simulink model "wlan_phy_tx_pmd"  (Simulink 7.8)
settings: Solver=ode45  StartTime=0.0  StopTime=17e3  RelTol=1e-3
PostLoadFcn:
  | wlan_phy_tx_init
InitFcn:
  | wlan_phy_tx_init
StartFcn:
  | wlan_phy_tx_init
values from neighbouring files (symbols this model uses):
  interleave_64QAM_addr = interleave_64QAM + 2*floor(interleave_64QAM/6)    [wlan_phy_tx_init.m]
  MAX_NUM_BYTES = 4096    [wlan_phy_tx_init.m]
  MAX_NUM_SC = 64    [wlan_phy_tx_init.m]
  Preamble_IQ = PLCP_Preamble.Preamble_t    [wlan_phy_tx_init.m]
undefined symbols (not defined in the file or in its folder): gcbh, interleave_16QAM, interleave_bpsk, interleave_QPSK, Mod_Constellation_16QAM, Mod_Constellation_64QAM, Mod_Constellation_BPSK, Mod_Constellation_QPSK, xlBlockLoadCallback, xlGetNormalizedPeriod
libraries: xbsIndex_r4 x1023, xbsEDKLib_r4 x1
(part 1 of 8)
settings Model: Creator=murphpo  LastModifiedBy=murphpo
settings DebuggingCC: SolverPrmCheckMsg=none  InheritedTsInSrcMsg=none  UnconnectedInputMsg=none  UnconnectedOutputMsg=none  UnconnectedLineMsg=none

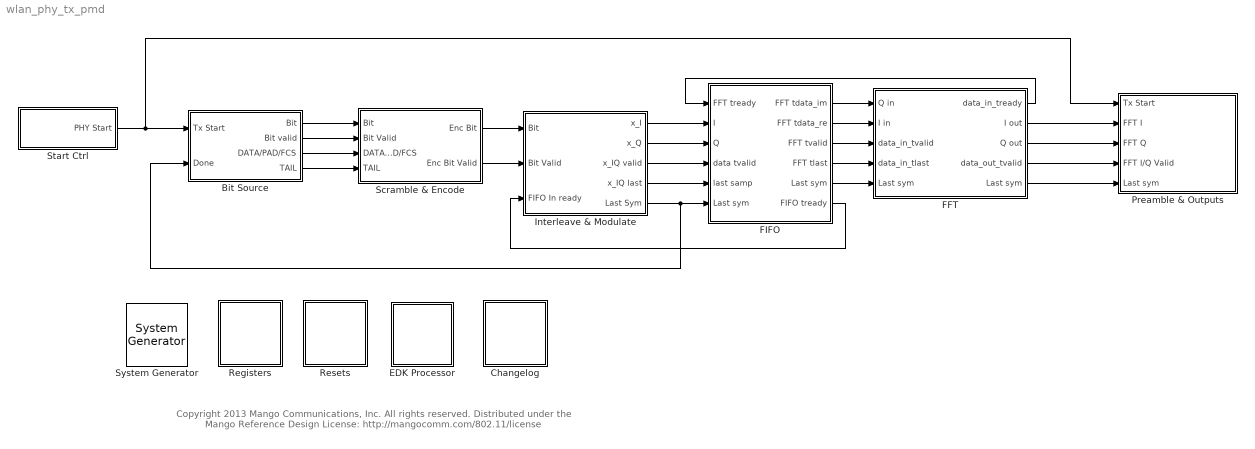
== system wlan_phy_tx_pmd ==
  note: Copyright 2013 Mango Communications, Inc. All rights reserved.
      |
      | Distributed under the Mango Reference Design License:
      | http://mangocomm.com/802.11/license
  " System Generator" : xbsIndex_r4/ System Generator  Tag=genX  xilinxfamily=virtex6  part=xc6vlx240t  speed=-2  package=ff1156  synthesis_tool=XST  clock_wrapper=Clock Enables  directory=./pcore_tx_v214  proj_type=Project Navigator  Synth_file=XST Defaults  Impl_file=ISE Defaults  testbench=off  simulink_period=1  sysclk_period=6.25  dcm_input_clock_period=10  incr_netlist=off  trim_vbits=Everywhere in SubSystem  dbl_ovrd=According to Block Masks  core_generation=According to Block Masks  run_coregen=off  deprecated_control=off  eval_field=0  block_type=sysgen
  Bit Source : Subsystem
  Changelog : Subsystem
  EDK Processor : Subsystem  LoadFcn=xlBlockLoadCallback(gcbh);  mask(Xilinx EDK Processor Block){mode=EDK pcore generation, xmp=, MemVisToProc=<qt bgcolor="#FFFFFF"><div><img src="S:/Xilinx/14.4/ISE_DS/ISE/sysgen/data/images/registerplus.gif"> &lt;&lt;Timing&gt;&gt;<br></div><div><img src="S:/Xilinx/14.4/ISE_DS/ISE/sysgen/data/images/registerplus.gif"> &lt;&lt;Config&gt;&gt;<br></div><div><img src="S:/Xilinx/14.4/ISE_DS/ISE/sysgen/data/images/registerplus.gif"> &lt;&lt;PKT_BUF_SEL&gt;&gt;<br></div><div><img src="S:/Xilinx/14.4/ISE_DS/ISE/sysgen/data/images/registerplus.gif"> &lt;&lt;Output_Scaling&gt;&gt;<br></div><div><img src="S:/Xilinx/14.4/ISE_DS/ISE/sysgen/data/images/registerplus.gif"> &lt;&lt;TX_START&gt;&gt;<br></div><div><img src="S:/Xilinx/14.4/ISE_DS/ISE/sysgen/data/images/registerplus.gif"> &lt;&lt;FFT_Config&gt;&gt;<br></div><div><img src="S:/Xilinx/14.4/ISE_DS/ISE/sysgen/data/images/registerplus.gif"> &lt;&lt;STATUS&gt;&gt;<br></div></qt>, AvailableMemories=<empty>, portInterfaceTable={'exposed'=>[],'portdir'=>[],'portname'=>[],'shortname'=>[]}, bus_type_sgadvanced=, bus_type=AXI, baseaddr=0x80000000, baseaddr_lock_sgadvanced=, baseaddr_lock=off, dual_clock_sgadvanced=, dual_clock=on, reg_readback_sgadvanced=, reg_readback=on, ucf_file=, inheritDeviceType_sgadvanced=, inheritDeviceType=off, elf_file=, codebug_sgadvanced=, codebug=on, clock_name=plb, internalPortList={}, resetPolarity=0, memxtable={'mladdr'=>[0.00000000000000000,1.00000000000000000,2.00000000000000000,3.00000000000000000,4.00000000000000000,5.00000000000000000,0.00000000000000000],'mlist'=>['wlan_phy_tx_pmd/Registers/From Register6','wlan_phy_tx_pmd/Registers/From Register5','wlan_phy_tx_pmd/Registers/From Register4','wlan_phy_tx_pmd/Registers/From Register3','wlan_phy_tx_pmd/Registers/From Register2','wlan_phy_tx_pmd/Registers/From Register1','wlan_phy_tx_pmd/Registers/To Register'],'mlname'=>['\\'Timing\\'','\\'Config\\'','\\'PKT_BUF_SEL\\'','\\'Output_Scaling\\'','\\'TX_START\\'','\\'FFT_Config\\'','\\'STATUS\\''],'mlstate'=>[0.00000000000000000,0.00000000000000000,0.00000000000000000,0.00000000000000000,0.00000000000000000,0.00000000000000000,0.00000000000000000]}, procinfo={}, memmapdirty=off, blockname=, xpsintstyle=default, has_advanced_control=0, sggui_pos=-1,-1,-1,-1, block_type=edkprocessor, block_version=2.7, sg_icon_stat=58,60,-1,-1,white,blue,0,07734,right,,[ ],[ ], sg_mask_display=|, sg_list_contents={'table'=>{'AvailableMemories'=>'popup(<empty>)'}}, sg_blockgui_xml=}
      mask sg_mask_display=|
      | fprintf('','COMMENT: begin icon graphics');
      | patch([0 58 58 0 0 ],[0 0 60 60 0 ],[0.77 0.82 0.91 ]);
      | plot([0 58 58 0 0 ],[0 0 60 60 0 ]);
      | patch([11.2 22.76 30.76 38.76 46.76 30.76 19.2 11.2 ],[38.88 38.88 46.88 38.88 46.88 46.88 46.88 38.88 ],[1 1 1 ]);
      | patch([19.2 30.76 22.76 11.2 19.2 ],[30.88 30.88 38.88 38.88 30.88 ],[0.931 0.946 0.973 ]);
      | patch([11.2 22.76 30.76 19.2 11.2 ],[22.88 22.88 30.88 30.88 22.88 ],[1 1 1 ]);
      | patch([19.2 46.76 38.76 30.76 22.76 11.2 19.2 ],[14.88 14.88 22.88 14.88 22.88 22.88 14.88 ],[0.931 0.946 0.973 ]);
      | fprintf('','COMMENT: end icon graphics');
      | fprintf('','COMMENT: begin icon text');
      | fprintf('','COMMENT: end icon text');
      mask prompts: mode "Configure Processor for"; xmp "XPS Project"; MemVisToProc ""; AvailableMemories "Available Memories"; portInterfaceTable ""; bus_type_sgadvanced ""; bus_type "Bus Type"; baseaddr "Base Address"; baseaddr_lock_sgadvanced ""; baseaddr_lock "Lock"; dual_clock_sgadvanced ""; dual_clock "Dual Clocks"; reg_readback_sgadvanced ""; reg_readback "Register Read-Back"; ucf_file "Constraint File"; inheritDeviceType_sgadvanced ""; inheritDeviceType "Inherit Device Type"; elf_file "Initial Program"; codebug_sgadvanced ""; codebug "Enable Co-Debug with Xilinx SDK (Beta)"; clock_name ""; internalPortList ""; resetPolarity ""; memxtable ""; procinfo ""; memmapdirty ""; blockname ""; xpsintstyle ""; has_advanced_control ""; sggui_pos ""; block_type ""; block_version ""; sg_icon_stat ""; sg_mask_display ""; sg_list_contents ""; sg_blockgui_xml ""
      mask help: Xilinx EDK Processor
      mask init:
      | try
      |   tmp_gcb = gcb;
      |   tmp_gcbh = gcbh;
      |   if (strcmp('SysGenIndex',get_param(bdroot(tmp_gcbh),'tag')) && ~isempty(regexp(bdroot(tmp_gcb), '^xbs', 'once')))
      |     return;
      |   end;
      |   xlMungeMaskParams;
      | 
      |   block_type='edkprocessor';
      | 
      |   serialized_declarations = '{''block_type''=>''String''}';
      |   xledkprocessor_init();
      |   ptable_ = xlblockprep(get_param(tmp_gcb, 'MaskWSVariables'));
      |   try
      |     xlBlockMoveCallback(tmp_gcbh);
      |   catch 
      |      clear global xl_updateicon_recursion_guard;
      |   end;
      | catch
      |   global dbgsysgen;
      |   if(~isempty(dbgsysgen) && dbgsysgen)
      |     e = regexprep(lasterr, '\n', '\nError: ');
      |     disp(['Error: While running MaskInit code on block ' tmp_gcb ': ' e]);
      |     error(e);
      |   end
      | end
      settings: CopyFcn=xlProcBlockCopyCallback(gcbh);xlBlockMoveCallback(gcbh);  DeleteFcn=xlDestroyGui(gcbh);  ModelCloseFcn=xlDestroyGui(gcbh);  PreSaveFcn=xlBlockPreSaveCallback(gcbh);  PostSaveFcn=xlBlockPostSaveCallback(gcbh);  DestroyFcn=xlDestroyGui(gcbh);  OpenFcn=bh=gcbh;xlProcBlockCallbacks('populatesharedmemorylistbox',bh);xlOpenGui(bh, 'edkprocessor_gui.xml', @xlProcBlockEnablement, @xlProcBlockAction);  CloseFcn=xlDestroyGui(gcbh);  MoveFcn=xlBlockMoveCallback(gcbh);
      mask Help: eval('');xlDoc('-book','sysgen','-topic','EDK_Processor');
      mask StyleString: popup(EDK pcore generation|HDL netlisting),edit,edit,edit,edit,edit,popup(AXI|PLB),edit,edit,checkbox,edit,checkbox,edit,checkbox,edit,edit,checkbox,edit,edit,checkbox,edit,edit,edit,edit,edit,edit,edit,edit,edit,edit,edit,edit,edit,edit,edit,edit
      mask Display:
      | fprintf('','COMMENT: begin icon graphics');
      | patch([0 58 58 0 0 ],[0 0 60 60 0 ],[0.77 0.82 0.91 ]);
      | plot([0 58 58 0 0 ],[0 0 60 60 0 ]);
      | patch([11.2 22.76 30.76 38.76 46.76 30.76 19.2 11.2 ],[38.88 38.88 46.88 38.88 46.88 46.88 46.88 38.88 ],[1 1 1 ]);
      | patch([19.2 30.76 22.76 11.2 19.2 ],[30.88 30.88 38.88 38.88 30.88 ],[0.931 0.946 0.973 ]);
      | patch([11.2 22.76 30.76 19.2 11.2 ],[22.88 22.88 30.88 30.88 22.88 ],[1 1 1 ]);
      | patch([19.2 46.76 38.76 30.76 22.76 11.2 19.2 ],[14.88 14.88 22.88 14.88 22.88 22.88 14.88 ],[0.931 0.946 0.973 ]);
      | fprintf('','COMMENT: end icon graphics');
      | fprintf('','COMMENT: begin icon text');
      | disp('');
      | 
      | fprintf('','COMMENT: end icon text');
  FFT : Subsystem
  FIFO : Subsystem
  Interleave & Modulate : Subsystem
  Preamble & Outputs : Subsystem
  Registers : Subsystem
  Resets : Subsystem
  Scramble & Encode : Subsystem
  Start Ctrl : Subsystem
  wires:
  Scramble & Encode/1(Enc Bit) -> Interleave & Modulate/1(Bit)
  Scramble & Encode/2(Enc Bit Valid) -> Interleave & Modulate/2(Bit Valid)
  Bit Source/1(Bit) -> Scramble & Encode/1(Bit)
  Bit Source/2(Bit valid) -> Scramble & Encode/2(Bit Valid)
  Bit Source/3(DATA/PAD/FCS) -> Scramble & Encode/3(DATA/PAD/FCS)
  Start Ctrl/1(PHY Start) -> Bit Source/1(Tx Start), Preamble & Outputs/1(Tx Start)
  Interleave & Modulate/1(x_I) -> FIFO/2(I)
  Interleave & Modulate/2(x_Q) -> FIFO/3(Q)
  Interleave & Modulate/3(x_IQ valid) -> FIFO/4(data tvalid)
  Interleave & Modulate/4(x_IQ last) -> FIFO/5(last samp)
  FIFO/4(FFT tlast) -> FFT/4(data_in_tlast)
  FIFO/1(FFT tdata_im) -> FFT/1(Q in)
  FIFO/2(FFT tdata_re) -> FFT/2(I in)
  FIFO/3(FFT tvalid) -> FFT/3(data_in_tvalid)
  FFT/1(data_in_tready) -> FIFO/1(FFT tready)
  FIFO/6(FIFO tready) -> Interleave & Modulate/3(FIFO In ready)
  Bit Source/4(TAIL) -> Scramble & Encode/4(TAIL)
  Interleave & Modulate/5(Last Sym) -> FIFO/6("Last sym "), Bit Source/2(Done)
  FIFO/5(Last sym) -> FFT/5("Last sym ")
  FFT/2(I out) -> Preamble & Outputs/2(FFT I)
  FFT/3(Q out) -> Preamble & Outputs/3(FFT Q)
  FFT/4(data_out_tvalid) -> Preamble & Outputs/4(FFT I/Q Valid)
  FFT/5(Last sym) -> Preamble & Outputs/5(Last sym)

== system wlan_phy_tx_pmd/Bit Source ==
  Tx Start : Inport
  Done : Inport  Port=2
  Addr Gen : Subsystem
  BRAM IF 64b : Subsystem
  Bit Per Sym Counter : Subsystem
  Bit Src : Scope  NumInputPorts=7
      settings: TimeRange=10000  YMin=-1~-1~0~0~8800~0~0  YMax=1~1~1~1~10400~1~1  SaveName=ScopeData2
  Data Sel 64b : Subsystem
  Delay{,1..6} (7 alike) : xbsIndex_r4/Delay  rst=off  infoeditControl=Selection of Reset will increase slice count due to use of real FFs and instead of SRLs  en=off  latency=1  dbl_ovrd=off  reg_retiming=off  block_type=delay
  Gateway Out{1..6,8} (7 alike) : xbsIndex_r4/Gateway Out  inherit_from_input=off  hdl_port=off  timing_constraint=None  locs_specified=off  LOCs={}  UseAsDAC=off  DACChannel='1'  block_type=gatewayout
  Logical1 : xbsIndex_r4/Logical  logical_function=OR  inputs=3  en=off  latency=0  precision=Full  arith_type=Unsigned  n_bits=16  bin_pt=0  align_bp=on  dbl_ovrd=off  block_type=logical
  Logical2 : xbsIndex_r4/Logical  logical_function=OR  inputs=2  en=off  latency=0  precision=Full  arith_type=Unsigned  n_bits=16  bin_pt=0  align_bp=on  dbl_ovrd=off  block_type=logical
  Logical3 : xbsIndex_r4/Logical  logical_function=OR  inputs=2  en=off  latency=0  precision=Full  arith_type=Unsigned  n_bits=16  bin_pt=0  align_bp=on  dbl_ovrd=off  block_type=logical
  Posedge : Subsystem
  S-R Latch : Subsystem
  SIGNAL Capture : Subsystem
  Sym Compute Ctrl : Subsystem
  Bit : Outport
  Bit valid : Outport  Port=2
  DATA/PAD/FCS : Outport  Port=3
  TAIL : Outport  Port=4
  tag scope: SIGNAL_DECODE_ERROR=global
  wires:
  Delay1/1 -> Data Sel 64b/2(Bit Ind)
  Delay/1 -> Bit valid/1, Gateway Out6/1, Data Sel 64b/6(RAM Valid)
  Posedge/1(Q) -> S-R Latch/1(S)
  S-R Latch/1(Q) -> Sym Compute Ctrl/1(Tx Running)
  Tx Start/1 -> Posedge/1(D), Gateway Out8/1
  Addr Gen/1(Bit Mem Addr) -> Delay1/1, BRAM IF 64b/1(Bit Addr), Gateway Out4/1
  Addr Gen/2(DATA) -> Delay2/1
  Delay2/1 -> Logical1/1, Data Sel 64b/5(DATA)
  Addr Gen/6(SIGNAL) -> Delay3/1
  SIGNAL Capture/1(Error) -> [SIGNAL_DECODE_ERROR]
  Delay3/1 -> SIGNAL Capture/2(En)
  Bit Per Sym Counter/1(Load Bit) -> Addr Gen/1(en), Delay/1, Gateway Out3/1
  Logical2/1 -> S-R Latch/2(R), Gateway Out1/1
  Sym Compute Ctrl/1(Start Next Sym) -> Bit Per Sym Counter/1(Start Sym), Gateway Out2/1
  Bit Per Sym Counter/2(Last Bit in Sym) -> Sym Compute Ctrl/2(Last Bit in Sym)
  Addr Gen/3(FCS) -> Delay5/1
  Addr Gen/4(TAIL) -> Delay4/1
  Delay5/1 -> Logical1/3, Data Sel 64b/3(FCS)
  Gateway Out8/1 -> Bit Src/1  "Tx Start"
  Gateway Out1/1 -> Bit Src/2  "Reset"
  Gateway Out2/1 -> Bit Src/3  "Start Sym"
  Gateway Out3/1 -> Bit Src/4  "Load Bit"
  Gateway Out4/1 -> Bit Src/5  "Bit Addr"
  Gateway Out5/1 -> Bit Src/6  "Bit Out"
  Gateway Out6/1 -> Bit Src/7  "Bit Out Valid"
  Addr Gen/5(PAD) -> Delay6/1
  Delay6/1 -> Logical3/2, Logical1/2
  Delay4/1 -> Logical3/1, TAIL/1
  Logical3/1 -> Data Sel 64b/4(PAD/TAIL)
  Logical1/1 -> DATA/PAD/FCS/1
  [TX_RESET] -> Logical2/1
  Done/1 -> Logical2/2
  BRAM IF 64b/1(64b Data) -> Data Sel 64b/1(RAM 64b), SIGNAL Capture/1(Data)
  Data Sel 64b/1(b) -> Bit/1, Gateway Out5/1

== system wlan_phy_tx_pmd/Changelog ==
  note: 2.00.a:
      | -First export as _pmd, with I/O for mac_hw integration
      |
      | 2.00.b:
      | -Changed pkt buf interface to 64b
      | -Added pkt buf addr offset
      |
      | 2.00.c:
      | -Fixed puncturing timing
      | -Enabled BPSK/QPSK 3/4 schemes
      |
      | 2.00.d:
      | -Attempting fix of bad pkt Tx (based on wireshark Rx checksum)
      |   at 3/4; suspected bug in not puncturing TAIL
      |
      | 2.00.e:
      | -Reworked TxEn disable logic with programmable extension
      |   -Moved TX_END extension to new register
      |
      | 2.00.f:
      | -Added longer Tx -> Rx delay (250 cycles) to reduce RSSI/ADC
      |   transients at Rx post Tx
      |
      | 2.00.g:
      | -Added RX_SIGS_INVALID output to supress post-Tx transients from
      |   ADCs at input to PHY Rx
      |
      | 2.00.h:
      | -Added 16QAM support
      |   -64QAM is trickier; interleaver will need new arch, since 1->6 isn't a supported DPRAM aspect ratio
      |
      | 2.00.i:
      | -Added 64QAM support
      |
      | 2.00.j:
      | -Fixed slip-by-1-per-symbol bug in FFT start timing (broke long-duration pkts)
      | -Added reg bit to not reset scrambling LFSR per pkt
      |
      | 2.00.k:
      | -Added RF B DAC outputs; A/B selection done via config register
      |
      | 2.00.l:
      | -Fixed zero sample between preamble and first OFDM symbol
      | -Removed unused reset port
      |
      | 2.00.m:
      | -More output mux timing bug fixes (last sample of pkt was being dropped)
      |
      | 2.00.n:
      | -Added explicit DAC_TX_CLK input to replace upsampled T=8 constant as IQ clock enable
      | -Replaced delays with registers in preamble output delays
      | -Added (x || FORCE_RESET) to SR latches in start ctrl (trying to fix very rare perma-Tx mode on download)
      | -Added (x || posedge(tx_start)) to output FIFO reset (trying to fix very rare extra sample between LTS - SIGNAL)
